simulink model "RollReference"  (R2012b)
settings: configuration reference "configSetObj_autopilot" (kept outside this file)
libraries: simulink x1
settings Model: RecordCoverage=on  Creator=ssauvage  LastModifiedBy=ssauvage

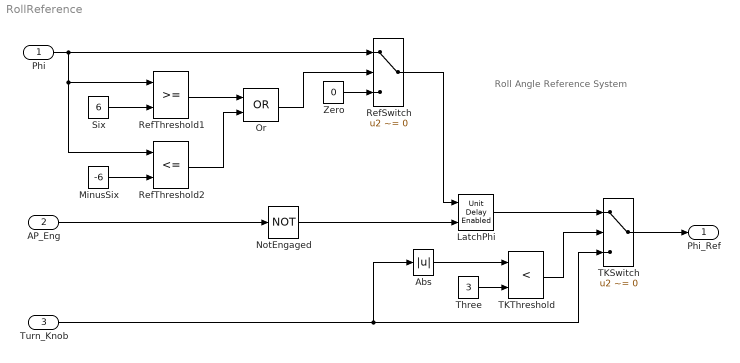
== system RollReference ==
  note: Roll Angle Reference
      | System
  Phi : Inport  RequirementInfo={} %GIDa_c3a462d2_08b4_4e77_8c2d_54dbbf10ff84
  AP_Eng : Inport  RequirementInfo={} %GIDa_eab3cf5e_076a_43af_9526_248eb18a4600  Port=2  OutDataTypeStr=boolean
  Turn_Knob : Inport  RequirementInfo={} %GIDa_390b9f48_ad7f_4348_b724_383349fea471  Port=3
  Abs : Abs  RequirementInfo={} %GIDa_ffb72df7_e3ee_4161_8a15_9dac0b2e2111
  LatchPhi : simulink/Additional Math & Discrete/Additional Discrete/Unit Delay Enabled  RequirementInfo={} %GIDa_8c0d03f6_d5c5_402f_aa39_965edf828326  vinit=0.0  tsamp=1/40
  MinusSix : Constant  RequirementInfo={} %GIDa_5c74b9d0_9c6f_4b63_8684_f8ff7492a869  Value=-6
  NotEngaged : Logic  RequirementInfo={} %GIDa_65fed7fb_3ebf_4130_b8df_4349b366d80b  Operator=NOT  IconShape=distinctive  AllPortsSameDT=off  OutDataTypeStr=boolean
  Or : Logic  RequirementInfo={} %GIDa_bf952eac_79b7_4caa_bb98_39296aec27cd  Operator=OR  OutDataTypeStr=boolean
  RefSwitch : Switch  RequirementInfo={} %GIDa_09c84777_a96c_48f2_9b6b_0741c21d931c  Criteria=u2 ~= 0
  RefThreshold1 : RelationalOperator  RequirementInfo={} %GIDa_38c79a16_7b66_4688_84a4_9cf044d10da6  OutDataTypeStr=boolean  InputSameDT=on
  RefThreshold2 : RelationalOperator  RequirementInfo={} %GIDa_e1c027b7_38b1_4555_bc4c_729f017b461c  Operator=<=  OutDataTypeStr=boolean  InputSameDT=on
  Six : Constant  RequirementInfo={} %GIDa_1e1bafb0_eb4b_4b23_92fd_3784c7f008c3  Value=6
  TKSwitch : Switch  RequirementInfo={} %GIDa_0d87cb36_522c_4438_9aa0_016f8591f195  Criteria=u2 ~= 0
  TKThreshold : RelationalOperator  RequirementInfo={} %GIDa_36c5c3a7_0f8c_4fff_adef_86046ce62a2b  Operator=<  OutDataTypeStr=boolean  InputSameDT=on
  Three : Constant  RequirementInfo={} %GIDa_790355a0_9e2a_4e09_aa99_5469577da1fe  Value=3  OutDataTypeStr=double
  Zero : Constant  RequirementInfo={} %GIDa_4c5f8a19_c716_4636_8d98_49ea269a7ac3  Value=0
  Phi_Ref : Outport  RequirementInfo={} %GIDa_0b372fe5_6e52_44b2_9052_a3ac8c9c13a9
  wires:
  NotEngaged/1 -> LatchPhi/2
  RefSwitch/1 -> LatchPhi/1
  LatchPhi/1 -> TKSwitch/1
  TKThreshold/1 -> TKSwitch/2
  Turn_Knob/1 -> TKSwitch/3, Abs/1
  Three/1 -> TKThreshold/2
  Abs/1 -> TKThreshold/1
  Phi/1 -> RefSwitch/1, RefThreshold1/1, RefThreshold2/1
  AP_Eng/1 -> NotEngaged/1
  TKSwitch/1 -> Phi_Ref/1
  Six/1 -> RefThreshold1/2
  Zero/1 -> RefSwitch/3
  Or/1 -> RefSwitch/2
  RefThreshold1/1 -> Or/1
  RefThreshold2/1 -> Or/2
  MinusSix/1 -> RefThreshold2/2
